simulink model "Youbot"  (R2024b)
settings: Solver=FixedStepDiscrete  StartTime=0.0  StopTime=inf  FixedStep=0.01  RelTol=1e-3  EnableMultiTasking=on
values from neighbouring files (symbols this model uses):
  dt = (tf-ti)/n    (= 0.05)    [sss.m]    (also in youbotdynamiceqn.m = 0.1; youbotdynamiceqn_predefinedpath.m)
  Kd = 10    [youbotdynamiceqn.m]
  Kp = 10    [youbotdynamiceqn.m]
  L = 0.23    [sss.m]    (also in youbotdynamiceqn.m; youbotdynamiceqn_predefinedpath.m)
  M_r = [m  0  0 ... (first row only)    [sss.m]    (also in youbotdynamiceqn.m; youbotdynamiceqn_predefinedpath.m)
  M_w = diag([I_w1, I_w2, I_w3, I_w4])    [sss.m]    (also in youbotdynamiceqn.m; youbotdynamiceqn_predefinedpath.m)
  R = (1/r) * [  1, -1, -(L+l) ... (first row only)    [sss.m]    (also in youbotdynamiceqn.m; youbotdynamiceqn_predefinedpath.m)
  R_T = transpose(R)    [sss.m]    (also in youbotdynamiceqn.m; youbotdynamiceqn_predefinedpath.m)
undefined symbols (not defined in the file or in its folder): Angular, DiscIntNeverNeededParam, Linear
libraries: robotlib x2, mobileRoboticsLib x1
settings Model: SimulationMode=external  Creator=The MathWorks, Inc.  LastModifiedBy=a_met
settings SolverCC: AlgebraicLoopSolver=TrustRegion
settings DataIOCC: LimitDataPoints=on  SaveFormat=Array  ReturnWorkspaceOutputs=off
settings OptimizationCC: ZeroExternalMemoryAtStartup=off  ZeroInternalMemoryAtStartup=off  LifeSpan=1  MaxStackSize=64
settings DebuggingCC: SolverPrmCheckMsg=warning  UnconnectedInputMsg=warning  UnconnectedOutputMsg=warning  UnconnectedLineMsg=warning  SFUnexpectedBacktrackingDiag=warning  SFNoUnconditionalDefaultTransitionDiag=warning  SFExecutionAtInitializationDiag=none  ArithmeticOperatorsInVariantConditions=warning
settings HardwareCC: ProdBitPerPointer=32  ProdBitPerSizeT=32  ProdBitPerPtrDiffT=32  ProdLargestAtomicFloat=None  ProdIntDivRoundTo=Undefined  ProdEndianess=Unspecified  ProdWordSize=32  ProdHWDeviceType=Generic->Unspecified (assume 32-bit Generic)  TargetHWDeviceType=Generic->Unspecified (assume 32-bit Generic)  UseEmbeddedCoderFeatures=off
settings ModelReferenceCC: EnableRefExpFcnMdlSchedulingChecks=on  PropagateSignalLabelsOutOfModel=off
settings SFSimCC: SimUseLocalCustomCode=off  CustomCodeUndefinedFunction=UseInterfaceOnly  SimTargetLang=C++
settings RTWCC: Description=Embedded Coder  SystemTargetFile=ert.tlc  HardwareBoard=Robot Operating System (ROS)  TLCOptions=-aInlineSetEventsForThisBaseRateFcn=TLC_FALSE -aSuppressMultiTaskScheduler=TLC_FALSE -aRateBasedStepFcn=0  TemplateMakefile=ert_default_tmf  RTWUseLocalCustomCode=off  Toolchain=Catkin  TargetLang=C++  GPUComputeCapability=3.5
settings CodeAppCC: StateflowObjectComments=on
settings ERTTargetCC: MultiwordLength=2048  ERTCustomFileBanners=off  CodeInterfacePackaging=C++ class  SupportContinuousTime=on  SupportNonInlinedSFcns=on  RemoveResetFunc=off  SupportVariableSizeSignals=on  ModelStepFunctionPrototypeControlCompliant=off  InlinedParameterPlacement=Hierarchical  RootIOFormat=Structure reference  ConvertIfToSwitch=off  SuppressUnreachableDefaultCases=off  DynamicArrayContainerType=coder::array
settings ConfigComp: CovMetricSettings=dw  CovSaveCumulativeToWorkspaceVar=on  CovSaveSingleToWorkspaceVar=on  CovExternalEMLEnable=off  CovSFcnEnable=off

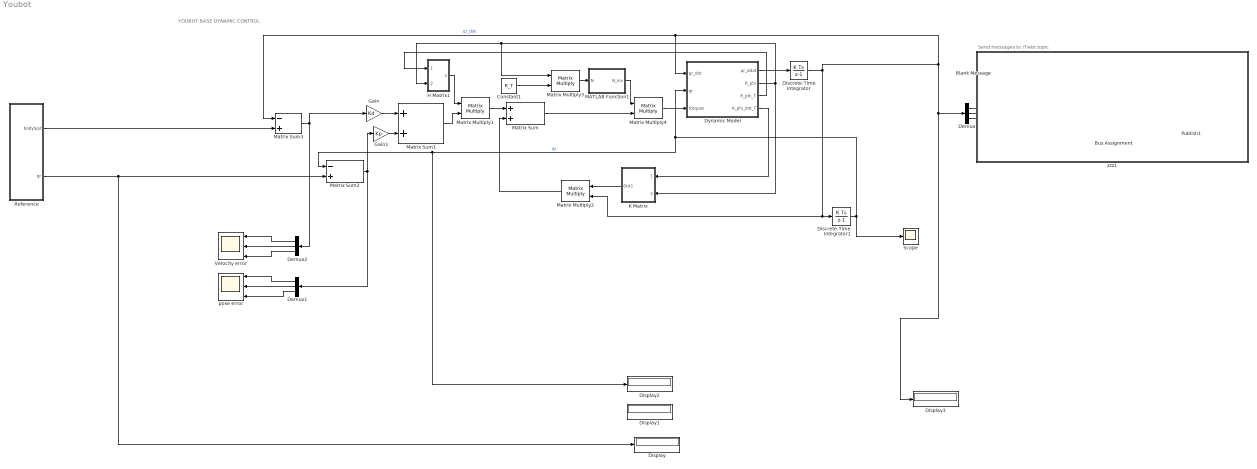
== system Youbot ==
  note: YOUBOT BASE DYNAMIC CONTROL
  note: Send messages to /Twist topic
  Blank Message : robotlib/Blank Message  messageClass=Message  entityType=geometry_msgs/Twist  messageType=geometry_msgs/Twist  SampleTime=inf  legacyBusStruct=off
  Bus Assignment : BusAssignment  AssignedSignals=Linear.X,Linear.Y,Angular.Z
  Constant1 : Constant  Value=R_T
  Demux : Demux  Outputs=3
  Demux1 : Demux  Outputs=3
  Demux2 : Demux  Outputs=3
  Discrete-Time Integrator : DiscreteIntegrator  SampleTime=-1  ICPrevOutput=DiscIntNeverNeededParam  ICPrevScaledInput=DiscIntNeverNeededParam
  Discrete-Time Integrator1 : DiscreteIntegrator  SampleTime=-1  ICPrevOutput=DiscIntNeverNeededParam  ICPrevScaledInput=DiscIntNeverNeededParam
  Display{,1..3} (4 alike) : Display
  Dynamic Model : Subsystem
  Gain : Gain  Gain=Kd
  Gain1 : Gain  Gain=Kp
  H Matrix1 : Subsystem
  K Matrix : Subsystem
  MATLAB Function1 : MATLAB Function  TreatAsAtomicUnit=on
  Matrix Sum : Sum
  Matrix Sum1 : Sum
  Matrix Sum2 : Sum  Inputs=-+
  Matrix Sum3 : Sum  Inputs=-+
  Matrix Multiply{1..4} (4 alike) : Product  Multiplication=Matrix(*)  SampleTime=dt
  Publish1 : robotlib/Publish  topicSource=Select from ROS network  topic=/cmd_vel  messageType=geometry_msgs/Twist  legacyBusStruct=off  messageQueueLength=105
  Reference : Subsystem
  Scope : Scope
  Velocity error : Scope  NumInputPorts=3
  pose error : Scope  NumInputPorts=3
  zzz1 : Subsystem  TreatAsAtomicUnit=on
      settings: OpenFcn=% no-op
      mask Display: disp('')
  wires:
  Bus Assignment/1 -> Publish1/1
  Blank Message/1 -> Bus Assignment/1
  Demux/1 -> Bus Assignment/2
  Demux/2 -> Bus Assignment/3
  Demux/3 -> Bus Assignment/4
  Gain1/1 -> Matrix Sum1/2
  Matrix Sum/1 -> Matrix Multiply4/2
  Discrete-Time Integrator1/1 -> Dynamic Model/2(qr), Matrix Sum2/1, Display2/1, Scope/1  "qr"
  Matrix Sum3/1 -> Demux2/1, Gain/1
  Matrix Multiply4/1 -> Dynamic Model/3(torques)
  H Matrix1/1(Out1) -> Matrix Multiply1/1
  Demux2/1 -> Velocity error/1
  Dynamic Model/4(R_phi_dot_T) -> K Matrix/1(R_phi_dot_T)
  Demux1/2 -> pose error/2
  Reference/2(qr) -> Display/1, Matrix Sum2/2
  Dynamic Model/3(R_phi_T) -> H Matrix1/1(R_phi_T)
  MATLAB Function1/1(N_inv) -> Matrix Multiply4/1
  Demux1/3 -> pose error/3
  Matrix Sum2/1 -> Demux1/1, Gain1/1
  Dynamic Model/1(qr_ddot) -> Discrete-Time Integrator/1
  Reference/1(bodySpd) -> Matrix Sum3/2
  Matrix Multiply1/1 -> Matrix Sum/1
  Demux2/3 -> Velocity error/3
  Matrix Sum1/1 -> Matrix Multiply1/2
  K Matrix/1(Out1) -> Matrix Multiply2/1
  Matrix Multiply3/1 -> MATLAB Function1/1(N)
  Discrete-Time Integrator/1 -> Discrete-Time Integrator1/1, Matrix Multiply2/2, Display3/1, Demux/1, Dynamic Model/1(qr_dot), Matrix Sum3/1  "qr_dot"
  Demux2/2 -> Velocity error/2
  Demux1/1 -> pose error/1
  Matrix Multiply2/1 -> Matrix Sum/2
  Gain/1 -> Matrix Sum1/1
  Constant1/1 -> Matrix Multiply3/2
  Dynamic Model/2(R_phi) -> K Matrix/2(R_phi_T), Matrix Multiply3/1, H Matrix1/2(R_phi)

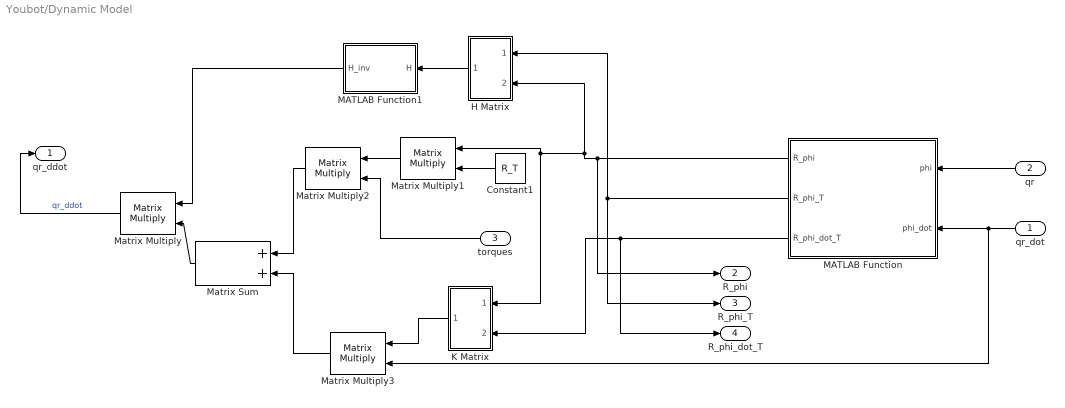
== system Youbot/Dynamic Model ==
  qr_dot : Inport
  qr : Inport  Port=2
  torques : Inport  Port=3
  Constant1 : Constant  Value=R_T
  H Matrix : Subsystem
  K Matrix : Subsystem
  MATLAB Function : MATLAB Function  TreatAsAtomicUnit=on
  MATLAB Function1 : MATLAB Function  TreatAsAtomicUnit=on
  Matrix Sum : Sum
  Matrix Multiply{,1..3} (4 alike) : Product  Multiplication=Matrix(*)  SampleTime=dt
  qr_ddot : Outport  PortDimensions=[3 1]
  R_phi : Outport  Port=2
  R_phi_T : Outport  Port=3
  R_phi_dot_T : Outport  Port=4
  wires:
  torques/1 -> Matrix Multiply2/2
  MATLAB Function/3(R_phi_dot_T) -> R_phi_dot_T/1, K Matrix/2(R_phi_dot_T)
  MATLAB Function/2(R_phi_T) -> R_phi_T/1, H Matrix/1(In2)
  qr_dot/1 -> Matrix Multiply3/2, MATLAB Function/2(phi_dot)
  Matrix Multiply2/1 -> Matrix Sum/1
  Matrix Multiply3/1 -> Matrix Sum/2
  K Matrix/1(Out1) -> Matrix Multiply3/1
  MATLAB Function1/1(H_inv) -> Matrix Multiply/1
  MATLAB Function/1(R_phi) -> R_phi/1, H Matrix/2(In1), Matrix Multiply1/1, K Matrix/1(R_phi)
  Constant1/1 -> Matrix Multiply1/2
  Matrix Multiply1/1 -> Matrix Multiply2/1
  qr/1 -> MATLAB Function/1(phi)
  Matrix Multiply/1 -> qr_ddot/1  "qr_ddot"
  Matrix Sum/1 -> Matrix Multiply/2
  H Matrix/1(Out1) -> MATLAB Function1/1(H)

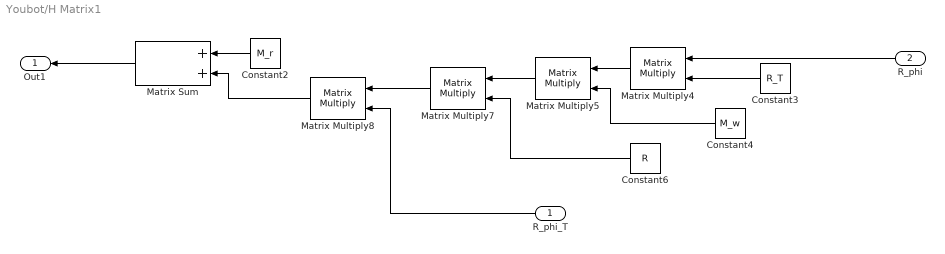
== system Youbot/H Matrix1 ==
  R_phi_T : Inport
  R_phi : Inport  Port=2
  Constant2 : Constant  Value=M_r
  Constant3 : Constant  Value=R_T
  Constant4 : Constant  Value=M_w
  Constant6 : Constant  Value=R
  Matrix Sum : Sum
  Matrix Multiply{4..5,7..8} (4 alike) : Product  Multiplication=Matrix(*)  SampleTime=dt
  Out1 : Outport
  wires:
  Constant2/1 -> Matrix Sum/1
  Matrix Multiply4/1 -> Matrix Multiply5/1
  R_phi_T/1 -> Matrix Multiply8/2
  Matrix Multiply7/1 -> Matrix Multiply8/1
  Constant6/1 -> Matrix Multiply7/2
  Matrix Multiply8/1 -> Matrix Sum/2
  Constant4/1 -> Matrix Multiply5/2
  Constant3/1 -> Matrix Multiply4/2
  Matrix Sum/1 -> Out1/1
  Matrix Multiply5/1 -> Matrix Multiply7/1
  R_phi/1 -> Matrix Multiply4/1

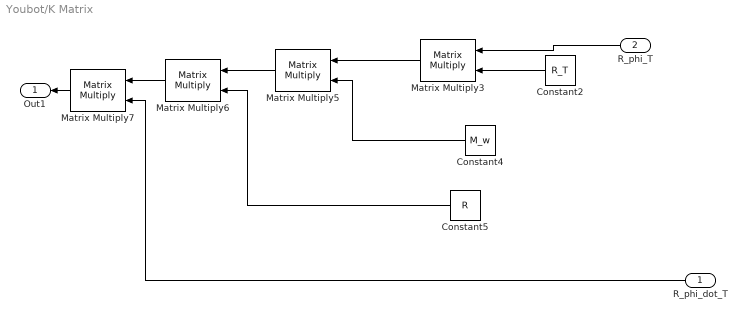
== system Youbot/K Matrix ==
  R_phi_dot_T : Inport
  R_phi_T : Inport  Port=2
  Constant2 : Constant  Value=R_T
  Constant4 : Constant  Value=M_w
  Constant5 : Constant  Value=R
  Matrix Multiply{3,5..7} (4 alike) : Product  Multiplication=Matrix(*)  SampleTime=dt
  Out1 : Outport  PortDimensions=[3 3]
  wires:
  Matrix Multiply7/1 -> Out1/1
  Matrix Multiply6/1 -> Matrix Multiply7/1
  Matrix Multiply3/1 -> Matrix Multiply5/1
  R_phi_T/1 -> Matrix Multiply3/1
  Constant4/1 -> Matrix Multiply5/2
  Constant5/1 -> Matrix Multiply6/2
  R_phi_dot_T/1 -> Matrix Multiply7/2
  Constant2/1 -> Matrix Multiply3/2
  Matrix Multiply5/1 -> Matrix Multiply6/1

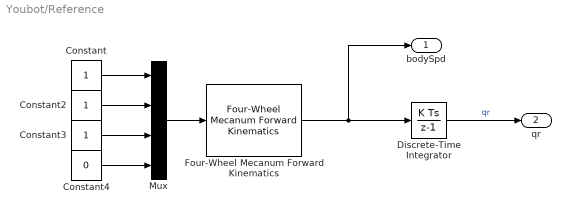
== system Youbot/Reference ==
  Constant : Constant
  Constant2 : Constant
  Constant3 : Constant
  Constant4 : Constant  Value=0
  Discrete-Time Integrator : DiscreteIntegrator  SampleTime=-1  ICPrevOutput=DiscIntNeverNeededParam  ICPrevScaledInput=DiscIntNeverNeededParam
  Four-Wheel Mecanum Forward Kinematics : mobileRoboticsLib/Kinematic Models/Four-Wheel Mecanum/Four-Wheel Mecanum Forward Kinematics  wheelRadius=r  wheelBase=2*L  wheelTrack=2*L
      settings: SourceProductName=Mobile Robotics Simulation Toolbox
  Mux : Mux
  bodySpd : Outport
  qr : Outport  Port=2
  wires:
  Constant2/1 -> Mux/2
  Constant4/1 -> Mux/4
  Constant3/1 -> Mux/3
  Discrete-Time Integrator/1 -> qr/1  "qr"
  Mux/1 -> Four-Wheel Mecanum Forward Kinematics/1
  Constant/1 -> Mux/1
  Four-Wheel Mecanum Forward Kinematics/1 -> Discrete-Time Integrator/1, bodySpd/1

== system Youbot/zzz1 ==

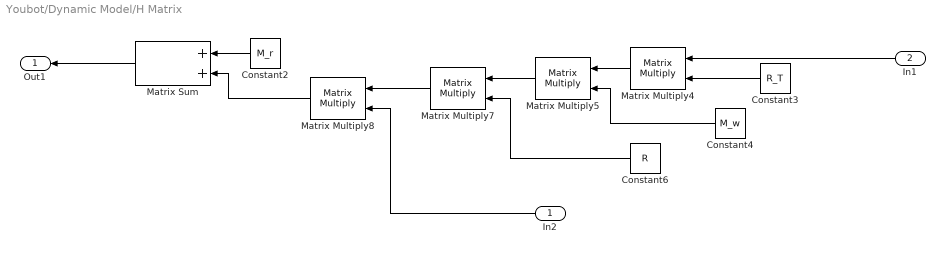
== system Youbot/Dynamic Model/H Matrix ==
  In2 : Inport
  In1 : Inport  Port=2
  Constant2 : Constant  Value=M_r
  Constant3 : Constant  Value=R_T
  Constant4 : Constant  Value=M_w
  Constant6 : Constant  Value=R
  Matrix Sum : Sum
  Matrix Multiply{4..5,7..8} (4 alike) : Product  Multiplication=Matrix(*)  SampleTime=dt
  Out1 : Outport
  wires:
  In1/1 -> Matrix Multiply4/1
  Matrix Multiply5/1 -> Matrix Multiply7/1
  Matrix Sum/1 -> Out1/1
  Constant3/1 -> Matrix Multiply4/2
  Constant4/1 -> Matrix Multiply5/2
  Matrix Multiply8/1 -> Matrix Sum/2
  Constant6/1 -> Matrix Multiply7/2
  Matrix Multiply7/1 -> Matrix Multiply8/1
  In2/1 -> Matrix Multiply8/2
  Matrix Multiply4/1 -> Matrix Multiply5/1
  Constant2/1 -> Matrix Sum/1

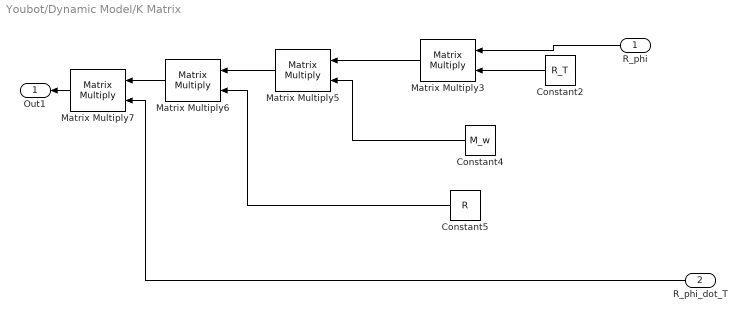
== system Youbot/Dynamic Model/K Matrix ==
  R_phi : Inport
  R_phi_dot_T : Inport  Port=2
  Constant2 : Constant  Value=R_T
  Constant4 : Constant  Value=M_w
  Constant5 : Constant  Value=R
  Matrix Multiply{3,5..7} (4 alike) : Product  Multiplication=Matrix(*)  SampleTime=dt
  Out1 : Outport
  wires:
  Matrix Multiply7/1 -> Out1/1
  Matrix Multiply6/1 -> Matrix Multiply7/1
  Matrix Multiply3/1 -> Matrix Multiply5/1
  R_phi/1 -> Matrix Multiply3/1
  Constant4/1 -> Matrix Multiply5/2
  Constant5/1 -> Matrix Multiply6/2
  R_phi_dot_T/1 -> Matrix Multiply7/2
  Constant2/1 -> Matrix Multiply3/2
  Matrix Multiply5/1 -> Matrix Multiply6/1

== matlab function Youbot/Dynamic Model/MATLAB Function1 ==
  data: H input; H_inv output
function H_inv = fcn(H)

H_inv = inv(H);

== matlab function Youbot/Dynamic Model/MATLAB Function ==
  data: phi input; R_phi output size=[3 3]; phi_dot input; R_phi_T output size=[3 3]; R_phi_dot_T output size=[3 3]
function [R_phi, R_phi_T, R_phi_dot_T] = fcn(phi, phi_dot)
    
    phi=phi(3);
    phi_dot=phi_dot(3);


    R_phi = [ cos(phi), -sin(phi), 0;
              sin(phi),  cos(phi), 0;
                    0  ,        0 , 1];

    R_phi_dot = [ -sin(phi)*phi_dot, -cos(phi)*phi_dot, 0;
                   cos(phi)*phi_dot,  -sin(phi)*phi_dot, 0;
                             0      ,              0    , 0];
    
    R_phi_T = transpose(R_phi);

    R_phi_dot_T = transpose(R_phi_dot)

end

== matlab function Youbot/MATLAB Function1 ==
  data: N input; N_inv output
function N_inv = fcn(N)

N_inv = pinv(N);
